simulink model "Pneumatic_act_PID"  (R2018b)
settings: Solver=ode15s  StartTime=0.0  StopTime=2  RelTol=5e-3
PreLoadFcn:
  | pneumaticInitialization
  | parametersMultibody
values from neighbouring files (symbols this model uses):
  base_breadth = 1    [parametersMultibody.m]
  base_height = 0.05    [parametersMultibody.m]
  base_length = 3.5    [parametersMultibody.m]
  box_breadth = 0.03    [parametersMultibody.m]
  box_height = 0.005    [parametersMultibody.m]
  box_height_s = 0.002    [parametersMultibody.m]
  box_length = 0.03    [parametersMultibody.m]
  box_yellow_breadth = 0.3    [parametersMultibody.m]
  box_yellow_height = 0.02    [parametersMultibody.m]
  box_yellow_length = 0.2    [parametersMultibody.m]
  frame_stand_breadth = 0.02    [parametersMultibody.m]
  frame_stand_height = 0.4280    (= 0.428)    [parametersMultibody.m]
  frame_stand_length = 0.02    [parametersMultibody.m]
undefined symbols (not defined in the file or in its folder): A_pipe, A_piston, delta_p, L_pipe, L_piston, p_init, sigbuilder_block, T_init, X, Y, Z
libraries: sm_lib x51, fl_lib x33, Contact_Forces_Lib x15, nesl_utility x7, simulink x2, Multibody_Parts_Lib x2, SimscapeFluids_lib x1, sm_backhoe_lib x1
(part 3 of 4)

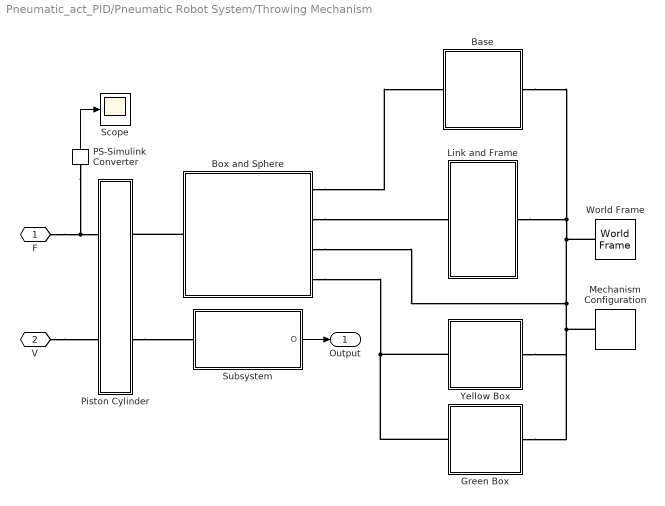
== system Pneumatic_act_PID/Pneumatic Robot System/Throwing Mechanism ==
  Base : Subsystem
      mask Display:
      | image("Base.jpg")
      | port_label('rconn', 1, 'B')
      | port_label('lconn', 1, 'W')
  Box and Sphere : Subsystem
      mask Display:
      | image('Box_ball.jpg')
      | port_label('rconn', 1, 'L')
      | port_label('lconn', 1, 'Base')
      | port_label('lconn', 2, 'Link_port')
      | port_label('lconn', 3, 'T')
      | port_label('lconn', 4, 'Ball_port')
  Green Box : Subsystem
      mask Display:
      | image("Box_green.jpg")
      | port_label('lconn', 1, 'BP')
      | port_label('rconn', 1, 'W')
  Link and Frame : Subsystem
      mask Display:
      | image('Frame_link.jpg')
      | port_label('rconn', 1, 'LP')
      | port_label('lconn', 1, 'T')
  Mechanism Configuration : sm_lib/Utilities/Mechanism Configuration  UniformGravity=Constant  GravityVector=[0 0 -9.80665]  GravityUnits=m/s^2  LinearizationDelta=0.001
  PS-Simulink Converter : nesl_utility/PS-Simulink Converter  PhysicalDomain=network_engine_domain  SubClassName=ps_output  LeftPortType=input  RightPortType=output  PseudoPeriodic=off  Frequencies=[]  Unit=1  AffineConversion=off
  Piston Cylinder : Subsystem
      mask Display: image('Piston_cyl.jpg')
  Scope : Scope
  Subsystem : Subsystem
  World Frame : sm_lib/Frames and Transforms/World Frame
  Yellow Box : Subsystem
      mask Display:
      | image("Box_yellow.jpg")
      | port_label('lconn', 1, 'BP')
      | port_label('rconn', 1, 'W')
  F : PMIOPort  Side=Left
  V : PMIOPort  Port=2  Side=Left
  Output : Outport
  wires:
  Subsystem/1(O) -> Output/1
  PS-Simulink Converter/1 -> Scope/1
  connections:
  Base/LConn1 -- World Frame/RConn1 -- Box and Sphere/LConn3 -- Mechanism Configuration/RConn1 -- Green Box/RConn1 -- Yellow Box/RConn1 -- Link and Frame/LConn1
  Box and Sphere/RConn1 -- Piston Cylinder/RConn1
  Green Box/LConn1 -- Box and Sphere/LConn4 -- Yellow Box/LConn1
  Box and Sphere/LConn2 -- Link and Frame/RConn1
  Box and Sphere/LConn1 -- Base/RConn1
  Piston Cylinder/RConn2 -- Subsystem/LConn1
  F/RConn1 -- Piston Cylinder/LConn1 -- PS-Simulink Converter/LConn1
  V/RConn1 -- Piston Cylinder/LConn2

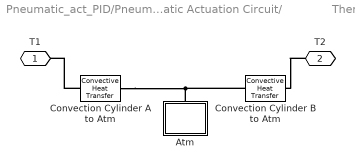
== system Pneumatic_act_PID/Pneumatic Robot System/Pneumatic Actuation Circuit/               Thermal Connection_3  ==
  Atm : Subsystem
      mask Display: disp('Atm')
  Convection Cylinder A to Atm : fl_lib/Thermal/Thermal Elements/Convective Heat Transfer  area=2*A_piston + sqrt(pi*A_piston)*L_piston m^2  heat_tr_coeff=20 W/(m^2 * K)  T_specify=off  T_priority=None  T=0 K  T_nominal_specify=off  T_nominal_unit=K  T_nominal_value=1  Q_specify=off  Q_priority=None  Q=0 W  Q_nominal_specify=off  Q_nominal_unit=W  Q_nominal_value=1
  Convection Cylinder B to Atm : fl_lib/Thermal/Thermal Elements/Convective Heat Transfer  area=2*A_piston + sqrt(pi*A_piston)*L_piston m^2  heat_tr_coeff=20 W/(m^2 * K)  T_specify=off  T_priority=None  T=0 K  T_nominal_specify=off  T_nominal_unit=K  T_nominal_value=1  Q_specify=off  Q_priority=None  Q=0 W  Q_nominal_specify=off  Q_nominal_unit=W  Q_nominal_value=1
  T1 : PMIOPort  Side=Left
  T2 : PMIOPort  Port=2  Side=Left
  connections:
  Convection Cylinder A to Atm/RConn1 -- Convection Cylinder B to Atm/RConn1 -- Atm/RConn1
  Convection Cylinder A to Atm/LConn1 -- T1/RConn1
  T2/RConn1 -- Convection Cylinder B to Atm/LConn1

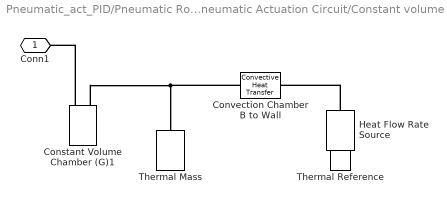
== system Pneumatic_act_PID/Pneumatic Robot System/Pneumatic Actuation Circuit/Constant volume chamber ==
  Constant Volume Chamber (G)1 : fl_lib/Gas/Elements/Constant Volume Chamber (G)  volume=volume m^3  area_A=area_A m^2  p_chamber_specify=on  p_chamber_priority=High  p_chamber=p_chamber MPa  p_chamber_nominal_specify=off  p_chamber_nominal_unit=MPa  p_chamber_nominal_value=1  T_chamber_specify=off  T_chamber_priority=High  T_chamber=293.15 K  T_chamber_nominal_specify=off  T_chamber_nominal_unit=K  T_chamber_nominal_value=1  rho_chamber_specify=off  rho_chamber_priority=None  rho_chamber=1.2 kg/m^3  rho_chamber_nominal_specify=off  rho_chamber_nominal_unit=kg/m^3  rho_chamber_nominal_value=1
      settings: SourceProductName=Simscape  SourceProductBaseCode=SS
  Convection Chamber B to Wall : fl_lib/Thermal/Thermal Elements/Convective Heat Transfer  area=area m^2  heat_tr_coeff=heat_tr_coeff W/(m^2 * K)  T_specify=off  T_priority=None  T=0 K  T_nominal_specify=off  T_nominal_unit=K  T_nominal_value=1  Q_specify=off  Q_priority=None  Q=0 W  Q_nominal_specify=off  Q_nominal_unit=W  Q_nominal_value=1
  Heat Flow Rate Source : fl_lib/Thermal/Thermal Sources/Heat Flow Rate Source  heat_flow=heat_flow W
      settings: SourceProductName=Simscape  SourceProductBaseCode=SS
  Thermal Mass : fl_lib/Thermal/Thermal Elements/Thermal Mass  mass=0.214 kg  sp_heat=840 J/kg/K  T_specify=on  T_priority=Low  T=293.15 K  T_nominal_specify=off  T_nominal_unit=K  T_nominal_value=1  Q_specify=off  Q_priority=None  Q=0 W  Q_nominal_specify=off  Q_nominal_unit=W  Q_nominal_value=1
  Thermal Reference : fl_lib/Thermal/Thermal Elements/Thermal Reference
  Conn1 : PMIOPort  Side=Left
  connections:
  Heat Flow Rate Source/LConn1 -- Convection Chamber B to Wall/LConn1
  Constant Volume Chamber (G)1/LConn2 -- Convection Chamber B to Wall/RConn1 -- Thermal Mass/LConn1
  Constant Volume Chamber (G)1/LConn1 -- Conn1/RConn1
  Thermal Reference/LConn1 -- Heat Flow Rate Source/RConn1

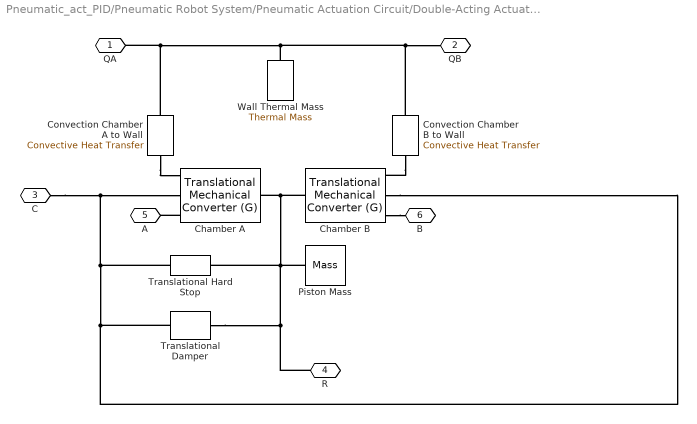
== system Pneumatic_act_PID/Pneumatic Robot System/Pneumatic Actuation Circuit/Double-Acting Actuator ==
  Chamber A : fl_lib/Gas/Elements/Translational Mechanical Converter (G)  mech_orientation=1  interface_area=A_piston m^2  length_init=x_init m  dead_volume=0.1 * A_piston * x_max m^3  area_A=A_port m^2  environment_spec=1  environment_pressure=0.101325 MPa  p_converter_specify=on  p_converter_priority=High  p_converter=p_init MPa  p_converter_nominal_specify=off  p_converter_nominal_unit=MPa  p_converter_nominal_value=1  T_converter_specify=on  T_converter_priority=High  T_converter=T_init K  T_converter_nominal_specify=off  T_converter_nominal_unit=K  T_converter_nominal_value=1  rho_converter_specify=off  rho_converter_priority=None  rho_converter=1.2 kg/m^3  rho_converter_nominal_specify=off  rho_converter_nominal_unit=kg/m^3  rho_converter_nominal_value=1
      settings: SourceProductName=Simscape  SourceProductBaseCode=SS
  Chamber B : fl_lib/Gas/Elements/Translational Mechanical Converter (G)  mech_orientation=-1  interface_area=A_piston m^2  length_init=- x_max + x_init m  dead_volume=0.1 * A_piston * x_max m^3  area_A=A_port m^2  environment_spec=1  environment_pressure=0.101325 MPa  p_converter_specify=on  p_converter_priority=High  p_converter=p_init MPa  p_converter_nominal_specify=off  p_converter_nominal_unit=MPa  p_converter_nominal_value=1  T_converter_specify=on  T_converter_priority=High  T_converter=T_init K  T_converter_nominal_specify=off  T_converter_nominal_unit=K  T_converter_nominal_value=1  rho_converter_specify=off  rho_converter_priority=None  rho_converter=1.2 kg/m^3  rho_converter_nominal_specify=off  rho_converter_nominal_unit=kg/m^3  rho_converter_nominal_value=1
      settings: SourceProductName=Simscape  SourceProductBaseCode=SS
  Convection Chamber A to Wall : fl_lib/Thermal/Thermal Elements/Convective Heat Transfer  area=2*A_piston + sqrt(pi*A_piston)*x_max m^2  heat_tr_coeff=heat_coeff W/(m^2 * K)  T_specify=off  T_priority=None  T=0 K  T_nominal_specify=off  T_nominal_unit=K  T_nominal_value=1  Q_specify=off  Q_priority=None  Q=0 W  Q_nominal_specify=off  Q_nominal_unit=W  Q_nominal_value=1
  Convection Chamber B to Wall : fl_lib/Thermal/Thermal Elements/Convective Heat Transfer  area=2*A_piston + sqrt(pi*A_piston)*x_max m^2  heat_tr_coeff=heat_coeff W/(m^2 * K)  T_specify=off  T_priority=None  T=0 K  T_nominal_specify=off  T_nominal_unit=K  T_nominal_value=1  Q_specify=off  Q_priority=None  Q=0 W  Q_nominal_specify=off  Q_nominal_unit=W  Q_nominal_value=1
  Piston Mass : fl_lib/Mechanical/Translational Elements/Mass  mass=M_piston kg  v_specify=off  v_priority=High  v=0 m/s  v_nominal_specify=off  v_nominal_unit=m/s  v_nominal_value=1  f_specify=off  f_priority=None  f=0 N  f_nominal_specify=off  f_nominal_unit=N  f_nominal_value=1
  Translational Damper : fl_lib/Mechanical/Translational Elements/Translational Damper  D=damp_mech N/(m/s)  v_specify=off  v_priority=None  v=0 m/s  v_nominal_specify=off  v_nominal_unit=m/s  v_nominal_value=1  f_specify=off  f_priority=None  f=0 N  f_nominal_specify=off  f_nominal_unit=N  f_nominal_value=1
  Translational Hard Stop : fl_lib/Mechanical/Translational Elements/Translational Hard Stop  upper_bnd=x_max m  lower_bnd=0 m  stiff_up=stiff_hard_stop N/m  stiff_low=stiff_hard_stop N/m  D_up=damp_hard_stop N/(m/s)  D_low=damp_hard_stop N/(m/s)  model=3  transition=0.1 mm  v_specify=off  v_priority=None  v=0 m/s  v_nominal_specify=off  v_nominal_unit=m/s  v_nominal_value=1  f_specify=off  f_priority=None  f=0 N  f_nominal_specify=off  f_nominal_unit=N  f_nominal_value=1  x_specify=on  x_priority=High  x=x_init m  x_nominal_specify=off  x_nominal_unit=m  x_nominal_value=1
  Wall Thermal Mass : fl_lib/Thermal/Thermal Elements/Thermal Mass  mass=M_actuator kg  sp_heat=cp J/kg/K  T_specify=on  T_priority=High  T=T_init K  T_nominal_specify=off  T_nominal_unit=K  T_nominal_value=1  Q_specify=off  Q_priority=None  Q=0 W  Q_nominal_specify=off  Q_nominal_unit=W  Q_nominal_value=1
  QA : PMIOPort  Side=Left
  QB : PMIOPort  Port=2  Side=Right
  C : PMIOPort  Port=3  Side=Left
  R : PMIOPort  Port=4  Side=Right
  A : PMIOPort  Port=5  Side=Left
  B : PMIOPort  Port=6  Side=Right
  connections:
  Chamber B/RConn1 -- R/RConn1 -- Translational Damper/LConn1 -- Piston Mass/LConn1 -- Translational Hard Stop/LConn1 -- Chamber A/RConn1
  Convection Chamber A to Wall/RConn1 -- QA/RConn1 -- Wall Thermal Mass/LConn1 -- Convection Chamber B to Wall/RConn1 -- QB/RConn1
  Translational Hard Stop/RConn1 -- Chamber B/LConn2 -- Translational Damper/RConn1 -- C/RConn1 -- Chamber A/LConn2
  Chamber A/LConn1 -- A/RConn1
  Chamber B/LConn1 -- B/RConn1
  Convection Chamber A to Wall/LConn1 -- Chamber A/LConn3
  Convection Chamber B to Wall/LConn1 -- Chamber B/LConn3

== system Pneumatic_act_PID/Pneumatic Robot System/Pneumatic Actuation Circuit/Pipe A ==
  Pipe (G) : fl_lib/Gas/Elements/Pipe (G)  length=L_pipe m  area=A_pipe m^2  Dh=2*sqrt(A_pipe/pi) m  length_add=0.1 * L_pipe m  roughness=15e-6 m  Re_lam=2000  Re_tur=4000  shape_factor=64  Nu_lam=3.66  p_pipe_specify=on  p_pipe_priority=Low  p_pipe=0.101325 MPa  p_pipe_nominal_specify=off  p_pipe_nominal_unit=MPa  p_pipe_nominal_value=1  T_pipe_specify=on  T_pipe_priority=Low  T_pipe=293.15 K  T_pipe_nominal_specify=off  T_pipe_nominal_unit=K  T_pipe_nominal_value=1  rho_pipe_specify=on  rho_pipe_priority=Low  rho_pipe=1.2 kg/m^3  rho_pipe_nominal_specify=off  rho_pipe_nominal_unit=kg/m^3  rho_pipe_nominal_value=1
      settings: SourceProductName=Simscape  SourceProductBaseCode=SS
  Wall Thermal Mass : fl_lib/Thermal/Thermal Elements/Thermal Mass  mass=rho_wall * A_pipe * L_pipe kg  sp_heat=cp_wall J/kg/K  T_specify=off  T_priority=High  T=T_init K  T_nominal_specify=off  T_nominal_unit=K  T_nominal_value=1  Q_specify=off  Q_priority=None  Q=0 W  Q_nominal_specify=off  Q_nominal_unit=W  Q_nominal_value=1
  B : PMIOPort  Side=Right
  A : PMIOPort  Port=2  Side=Left
  T : PMIOPort  Port=3  Side=Left
  connections:
  Pipe (G)/RConn1 -- B/RConn1
  A/RConn1 -- Pipe (G)/LConn1
  Pipe (G)/LConn2 -- Wall Thermal Mass/LConn1 -- T/RConn1

== system Pneumatic_act_PID/Pneumatic Robot System/Pneumatic Actuation Circuit/Pipe B ==
  Pipe (G) : fl_lib/Gas/Elements/Pipe (G)  length=L_pipe m  area=A_pipe m^2  Dh=2*sqrt(A_pipe/pi) m  length_add=0.1 * L_pipe m  roughness=15e-6 m  Re_lam=2000  Re_tur=4000  shape_factor=64  Nu_lam=3.66  p_pipe_specify=on  p_pipe_priority=Low  p_pipe=0.101325 MPa  p_pipe_nominal_specify=off  p_pipe_nominal_unit=MPa  p_pipe_nominal_value=1  T_pipe_specify=on  T_pipe_priority=Low  T_pipe=293.15 K  T_pipe_nominal_specify=off  T_pipe_nominal_unit=K  T_pipe_nominal_value=1  rho_pipe_specify=on  rho_pipe_priority=Low  rho_pipe=1.2 kg/m^3  rho_pipe_nominal_specify=off  rho_pipe_nominal_unit=kg/m^3  rho_pipe_nominal_value=1
      settings: SourceProductName=Simscape  SourceProductBaseCode=SS
  Wall Thermal Mass : fl_lib/Thermal/Thermal Elements/Thermal Mass  mass=rho_wall * A_pipe * L_pipe kg  sp_heat=cp_wall J/kg/K  T_specify=off  T_priority=High  T=T_init K  T_nominal_specify=off  T_nominal_unit=K  T_nominal_value=1  Q_specify=off  Q_priority=None  Q=0 W  Q_nominal_specify=off  Q_nominal_unit=W  Q_nominal_value=1
  B : PMIOPort  Side=Right
  T : PMIOPort  Port=2  Side=Left
  A : PMIOPort  Port=3  Side=Left
  connections:
  T/RConn1 -- Wall Thermal Mass/LConn1 -- Pipe (G)/LConn2
  A/RConn1 -- Pipe (G)/LConn1
  Pipe (G)/RConn1 -- B/RConn1

== system Pneumatic_act_PID/Pneumatic Robot System/Pneumatic Actuation Circuit/Return Pipe ==
  Pipe (G) : fl_lib/Gas/Elements/Pipe (G)  length=L_pipe m  area=A_pipe m^2  Dh=2*sqrt(A_pipe/pi) m  length_add=0.1 * L_pipe m  roughness=15e-6 m  Re_lam=2000  Re_tur=4000  shape_factor=64  Nu_lam=3.66  p_pipe_specify=off  p_pipe_priority=Low  p_pipe=0.101325 MPa  p_pipe_nominal_specify=off  p_pipe_nominal_unit=MPa  p_pipe_nominal_value=1  T_pipe_specify=off  T_pipe_priority=Low  T_pipe=293.15 K  T_pipe_nominal_specify=off  T_pipe_nominal_unit=K  T_pipe_nominal_value=1  rho_pipe_specify=off  rho_pipe_priority=Low  rho_pipe=1.2 kg/m^3  rho_pipe_nominal_specify=off  rho_pipe_nominal_unit=kg/m^3  rho_pipe_nominal_value=1
      settings: SourceProductName=Simscape  SourceProductBaseCode=SS
  Wall Thermal Mass : fl_lib/Thermal/Thermal Elements/Thermal Mass  mass=rho_wall * A_pipe * L_pipe kg  sp_heat=cp_wall J/kg/K  T_specify=off  T_priority=None  T=300 K  T_nominal_specify=off  T_nominal_unit=K  T_nominal_value=1  Q_specify=off  Q_priority=None  Q=0 W  Q_nominal_specify=off  Q_nominal_unit=W  Q_nominal_value=1
  B : PMIOPort  Side=Right
  T : PMIOPort  Port=2  Side=Left
  A : PMIOPort  Port=3  Side=Left
  connections:
  Pipe (G)/RConn1 -- B/RConn1
  A/RConn1 -- Pipe (G)/LConn1
  Pipe (G)/LConn2 -- Wall Thermal Mass/LConn1 -- T/RConn1

== system Pneumatic_act_PID/Pneumatic Robot System/Pneumatic Actuation Circuit/Supply Pipe ==
  Pipe (G) : fl_lib/Gas/Elements/Pipe (G)  length=L_pipe m  area=A_pipe m^2  Dh=2*sqrt(A_pipe/pi) m  length_add=0.1 * L_pipe m  roughness=15e-6 m  Re_lam=2000  Re_tur=4000  shape_factor=64  Nu_lam=3.66  p_pipe_specify=on  p_pipe_priority=Low  p_pipe=0.101325 MPa  p_pipe_nominal_specify=off  p_pipe_nominal_unit=MPa  p_pipe_nominal_value=1  T_pipe_specify=on  T_pipe_priority=Low  T_pipe=293.15 K  T_pipe_nominal_specify=off  T_pipe_nominal_unit=K  T_pipe_nominal_value=1  rho_pipe_specify=on  rho_pipe_priority=Low  rho_pipe=1.2 kg/m^3  rho_pipe_nominal_specify=off  rho_pipe_nominal_unit=kg/m^3  rho_pipe_nominal_value=1
      settings: SourceProductName=Simscape  SourceProductBaseCode=SS
  Wall Thermal Mass : fl_lib/Thermal/Thermal Elements/Thermal Mass  mass=rho_wall * A_pipe * L_pipe kg  sp_heat=cp_wall J/kg/K  T_specify=off  T_priority=Low  T=T_init K  T_nominal_specify=off  T_nominal_unit=K  T_nominal_value=1  Q_specify=off  Q_priority=None  Q=0 W  Q_nominal_specify=off  Q_nominal_unit=W  Q_nominal_value=1
  B : PMIOPort  Side=Right
  A : PMIOPort  Port=2  Side=Left
  T : PMIOPort  Port=3  Side=Left
  connections:
  T/RConn1 -- Wall Thermal Mass/LConn1 -- Pipe (G)/LConn2
  A/RConn1 -- Pipe (G)/LConn1
  Pipe (G)/RConn1 -- B/RConn1

== system Pneumatic_act_PID/Pneumatic Robot System/Pneumatic Actuation Circuit/Thermal Connection_1 ==
  Atm2 : Subsystem
      mask Display: disp('Atm')
  Convection Return to Atm : fl_lib/Thermal/Thermal Elements/Convective Heat Transfer  area=2*sqrt(pi*A_pipe) * L_pipe m^2  heat_tr_coeff=20 W/(m^2 * K)  T_specify=off  T_priority=None  T=0 K  T_nominal_specify=off  T_nominal_unit=K  T_nominal_value=1  Q_specify=off  Q_priority=None  Q=0 W  Q_nominal_specify=off  Q_nominal_unit=W  Q_nominal_value=1
  Convection Supply to Atm : fl_lib/Thermal/Thermal Elements/Convective Heat Transfer  area=2*sqrt(pi*A_pipe) * L_pipe m^2  heat_tr_coeff=20 W/(m^2 * K)  T_specify=off  T_priority=None  T=0 K  T_nominal_specify=off  T_nominal_unit=K  T_nominal_value=1  Q_specify=off  Q_priority=None  Q=0 W  Q_nominal_specify=off  Q_nominal_unit=W  Q_nominal_value=1
  T1 : PMIOPort  Side=Left
  T2 : PMIOPort  Port=2  Side=Left
  connections:
  Convection Supply to Atm/LConn1 -- T1/RConn1
  Convection Return to Atm/RConn1 -- Convection Supply to Atm/RConn1 -- Atm2/RConn1
  Convection Return to Atm/LConn1 -- T2/RConn1

== system Pneumatic_act_PID/Pneumatic Robot System/Pneumatic Actuation Circuit/Thermal Connection_2 ==
  Atm1 : Subsystem
      mask Display: disp('Atm')
  Convection Pipe A to Atm : fl_lib/Thermal/Thermal Elements/Convective Heat Transfer  area=2*sqrt(pi*A_pipe) * L_pipe m^2  heat_tr_coeff=20 W/(m^2 * K)  T_specify=off  T_priority=None  T=0 K  T_nominal_specify=off  T_nominal_unit=K  T_nominal_value=1  Q_specify=off  Q_priority=None  Q=0 W  Q_nominal_specify=off  Q_nominal_unit=W  Q_nominal_value=1
  Convection Pipe B to Atm : fl_lib/Thermal/Thermal Elements/Convective Heat Transfer  area=2*sqrt(pi*A_pipe) * L_pipe m^2  heat_tr_coeff=20 W/(m^2 * K)  T_specify=off  T_priority=None  T=0 K  T_nominal_specify=off  T_nominal_unit=K  T_nominal_value=1  Q_specify=off  Q_priority=None  Q=0 W  Q_nominal_specify=off  Q_nominal_unit=W  Q_nominal_value=1
  T1 : PMIOPort  Side=Left
  T2 : PMIOPort  Port=2  Side=Left
  connections:
  Convection Pipe B to Atm/RConn1 -- Convection Pipe A to Atm/RConn1 -- Atm1/RConn1
  Convection Pipe A to Atm/LConn1 -- T1/RConn1
  Convection Pipe B to Atm/LConn1 -- T2/RConn1

== system Pneumatic_act_PID/Pneumatic Robot System/Throwing Mechanism/Base ==
  " Base" : sm_lib/Body Elements/Solid  InertiaType=CalculateFromGeometry  Mass=1  MassUnits=kg  CenterOfMass=[0 0 0]  CenterOfMassUnits=m  MomentsOfInertia=[1 1 1]  MomentsOfInertiaUnits=kg*m^2  ProductsOfInertia=[0 0 0]  ProductsOfInertiaUnits=kg*m^2  BasedOnType=Density  Density=1000  DensityUnits=kg/m^3  DoExposeReferenceFrame=on  SerializedFrames=<Frames/>  GraphicType=FromGeometry  MarkerShape=Sphere  MarkerSize=10  GraphicVisPropType=SimpleVisualProperties  GraphicDiffuseColor=[0.8 1 0.8]  GraphicSpecularColor=[0.5 0.5 0.5 1.0]  GraphicAmbientColor=[0.15 0.15 0.15 1.0]  GraphicEmissiveColor=[0.0 0.0 0.0 1.0]  GraphicShininess=75  GraphicOpacity=1.0  GeometryShape=Brick  RectangleSize=[1 1]  RectangleSizeUnits=m  BrickDimensions=[base_length base_breadth base_height]  BrickDimensionUnits=m  CylinderRadius=0.008  CylinderRadiusUnits=m  CylinderLength=0.1  CylinderLengthUnits=m  SphereRadius=1  SphereRadiusUnits=m  EllipsoidRadii=[1 1 1]  EllipsoidRadiiUnits=m  ExtrusionCrossSection=[1 1; -1 1; -1 -1; 1 -1]  ExtrusionCrossSectionUnits=m  ExtrusionLength=1  ExtrusionLengthUnits=m  PolygonNumSides=3  PolygonOuterRadius=1  PolygonOuterRadiusUnits=m  ExtGeomFileType=STEP  ExtGeomFileUnits=m  RevolutionCrossSection=[1 1; 1 -1; 2 -1; 2 1]  RevolutionCrossSectionUnits=m  RevolutionExtent=Full  RevolutionAngle=180  RevolutionAngleUnits=deg
  Rigid Transform3 : sm_lib/Frames and Transforms/Rigid Transform  TranslationMethod=Cartesian  TranslationStandardOffset=0.25  TranslationLengthUnit=m  TranslationStandardAxis=-Z  TranslationCartesianOffset=[1.2 0 -0.25]  TranslationROffset=0  TranslationROffsetUnits=m  TranslationZOffset=0  TranslationZOffsetUnits=m  TranslationThetaOffset=0  TranslationThetaOffsetUnits=deg  RotationMethod=None  RotationAngleUnits=deg  RotationStandardAxis=+X  RotationAngle=90  RotationArbitraryAxis=[0 0 1]  FollAlignAxisA=+X  BaseAlignAxisA=+Y  FollAlignAxisB=+Y  BaseAlignAxisB=+Z  RotationSequenceAxes=FollowerAxes  RotationSequence=XYX  RotationSequenceAngles=[0 0 0]  RotationSequenceAnglesUnits=deg  RotationMatrix=[1 0 0; 0 1 0; 0 0 1]
  B : PMIOPort  Side=Left
  Base : PMIOPort  Port=2  Side=Right
  connections:
  Rigid Transform3/RConn1 -- Base/RConn1 -- " Base"/RConn1
  Rigid Transform3/LConn1 -- B/RConn1

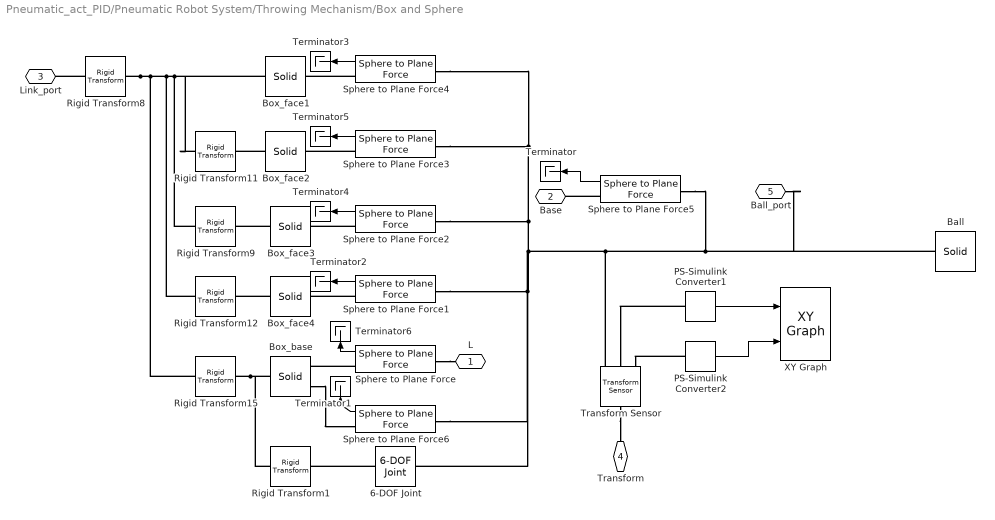
== system Pneumatic_act_PID/Pneumatic Robot System/Throwing Mechanism/Box and Sphere ==
  6-DOF Joint : sm_lib/Joints/6-DOF Joint  SenseConstraintForce=off  SenseConstraintForceX=off  SenseConstraintForceY=off  SenseConstraintForceZ=off  SenseConstraintTorque=off  SenseConstraintTorqueX=off  SenseConstraintTorqueY=off  SenseConstraintTorqueZ=off  SenseTotalForce=off  SenseTotalForceX=off  SenseTotalForceY=off  SenseTotalForceZ=off  SenseTotalTorque=off  SenseTotalTorqueX=off  SenseTotalTorqueY=off  SenseTotalTorqueZ=off  CompositeWrenchDir=FollowerOnBase  CompositeWrenchFrame=BaseFrame  PxEquilibriumPosition=0  PxEquilibriumPositionUnits=m  PxSpringStiffness=0  PxSpringStiffnessUnits=N/m  PxDampingCoefficient=0  PxDampingCoefficientUnits=N/(m/s)  PxTorqueActuationMode=NoTorque  PxMotionActuationMode=ComputedMotion  PxSensePosition=off  PxSenseVelocity=off  PxSenseAcceleration=off  PxSenseTorqueForce=off  PxPositionTargetSpecify=off  PxPositionTargetPriority=High  PxPositionTargetValue=0  PxPositionTargetValueUnits=m  PxVelocityTargetSpecify=off  PxVelocityTargetPriority=High  PxVelocityTargetValue=0  PxVelocityTargetValueUnits=m/s  PyEquilibriumPosition=0  PyEquilibriumPositionUnits=m  PySpringStiffness=0  PySpringStiffnessUnits=N/m  PyDampingCoefficient=0  PyDampingCoefficientUnits=N/(m/s)  PyTorqueActuationMode=NoTorque  PyMotionActuationMode=ComputedMotion  PySensePosition=off  PySenseVelocity=off  PySenseAcceleration=off  PySenseTorqueForce=off  PyPositionTargetSpecify=off  PyPositionTargetPriority=High  PyPositionTargetValue=0  PyPositionTargetValueUnits=m  PyVelocityTargetSpecify=off  PyVelocityTargetPriority=High  PyVelocityTargetValue=0  PyVelocityTargetValueUnits=m/s  PzEquilibriumPosition=0  PzEquilibriumPositionUnits=m  PzSpringStiffness=0  PzSpringStiffnessUnits=N/m  PzDampingCoefficient=0  PzDampingCoefficientUnits=N/(m/s)  PzTorqueActuationMode=NoTorque  PzMotionActuationMode=ComputedMotion  PzSensePosition=off  PzSenseVelocity=off  PzSenseAcceleration=off  PzSenseTorqueForce=off  PzPositionTargetSpecify=off  PzPositionTargetPriority=High  PzPositionTargetValue=0  PzPositionTargetValueUnits=m  PzVelocityTargetSpecify=off  PzVelocityTargetPriority=High  PzVelocityTargetValue=0  PzVelocityTargetValueUnits=m/s  SphDefPosRotationMethod=None  SphDefPosRotationAngleUnits=deg  SphDefPosRotationStandardAxis=+Z  SphDefPosRotationAngle=0.0  SphDefPosRotationArbitraryAxis=[0 0 1]  SphDefPosFollAlignAxisA=+X  SphDefPosBaseAlignAxisA=+Y  SphDefPosFollAlignAxisB=+Y  SphDefPosBaseAlignAxisB=+Z  SphDefPosRotationSequenceAxes=FollowerAxes  SphDefPosRotationSequence=XYX  SphDefPosRotationSequenceAngles=[0 0 0]  SphDefPosRotationSequenceAnglesUnits=deg  SphDefPosRotationMatrix=[1 0 0; 0 1 0; 0 0 1]  SphEqPosRotationMethod=None  SphEqPosRotationAngleUnits=deg  SphEqPosRotationStandardAxis=+Z  SphEqPosRotationAngle=0.0  SphEqPosRotationArbitraryAxis=[0 0 1]  SphEqPosFollAlignAxisA=+X  SphEqPosBaseAlignAxisA=+Y  SphEqPosFollAlignAxisB=+Y  SphEqPosBaseAlignAxisB=+Z  SphEqPosRotationSequenceAxes=FollowerAxes  SphEqPosRotationSequence=XYX  SphEqPosRotationSequenceAngles=[0 0 0]  SphEqPosRotationSequenceAnglesUnits=deg  SphEqPosRotationMatrix=[1 0 0; 0 1 0; 0 0 1]  SphSpringStiffness=0  SphSpringStiffnessUnits=N*m/deg  SphDampingCoefficient=1e-3  SphDampingCoefficientUnits=N*m/(rad/s)  SphActuateTorqueX=off  SphActuateTorqueY=off  SphActuateTorqueZ=off  SphActuateTorque=off  SphTorqueActuationMode=NoTorque  SphMotionActuationMode=ComputedMotion  SphActuationFrame=BaseFrame  SphSensePosition=off  SphSenseVelocityX=off  SphSenseVelocityY=off  SphSenseVelocityZ=off  SphSenseVelocity=off  SphSenseAccelerationX=off  SphSenseAccelerationY=off  SphSenseAccelerationZ=off  SphSenseAcceleration=off  SphSenseTorqueX=off  SphSenseTorqueY=off  SphSenseTorqueZ=off  SphSenseTorqueForce=off  SphSensingFrame=BaseFrame  SphPositionTargetRotationMethod=None  SphPositionTargetRotationAngleUnits=deg  SphPositionTargetRotationStandardAxis=+Z  SphPositionTargetRotationAngle=0.0  SphPositionTargetRotationArbitraryAxis=[0 0 1]  SphPositionTargetFollAlignAxisA=+X  SphPositionTargetBaseAlignAxisA=+Y  SphPositionTargetFollAlignAxisB=+Y  SphPositionTargetBaseAlignAxisB=+Z  SphPositionTargetRotationSequenceAxes=FollowerAxes  SphPositionTargetRotationSequence=XYX  SphPositionTargetRotationSequenceAngles=[0 0 0]  SphPositionTargetRotationSequenceAnglesUnits=deg  SphPositionTargetRotationMatrix=[1 0 0; 0 1 0; 0 0 1]  SphPositionTargetSpecify=off  SphPositionTargetPriority=High  SphVelocityTargetValue=[0 0 0]  SphVelocityTargetValueUnits=deg/s  SphVelocityTargetSpecify=off  SphVelocityTargetPriority=High  SphVelocityTargetInFollowerFrame=on
  Ball : sm_lib/Body Elements/Solid  InertiaType=CalculateFromGeometry  Mass=15  MassUnits=g  CenterOfMass=[0 0 0]  CenterOfMassUnits=m  MomentsOfInertia=[1 1 1]  MomentsOfInertiaUnits=kg*m^2  ProductsOfInertia=[0 0 0]  ProductsOfInertiaUnits=kg*m^2  BasedOnType=Density  Density=1000  DensityUnits=kg/m^3  DoExposeReferenceFrame=on  SerializedFrames=<Frames/>  GraphicType=FromGeometry  MarkerShape=Sphere  MarkerSize=10  GraphicVisPropType=SimpleVisualProperties  GraphicDiffuseColor=[1 1 0.4]  GraphicSpecularColor=[0.5 0.5 0.5 1.0]  GraphicAmbientColor=[0.15 0.15 0.15 1.0]  GraphicEmissiveColor=[0.0 0.0 0.0 1.0]  GraphicShininess=75  GraphicOpacity=1.0  GeometryShape=Sphere  RectangleSize=[1 1]  RectangleSizeUnits=m  BrickDimensions=[1 1 1]  BrickDimensionUnits=m  CylinderRadius=1  CylinderRadiusUnits=m  CylinderLength=1  CylinderLengthUnits=m  SphereRadius=radius_ball  SphereRadiusUnits=m  EllipsoidRadii=[1 1 1]  EllipsoidRadiiUnits=m  ExtrusionCrossSection=[1 1; -1 1; -1 -1; 1 -1]  ExtrusionCrossSectionUnits=m  ExtrusionLength=1  ExtrusionLengthUnits=m  PolygonNumSides=3  PolygonOuterRadius=1  PolygonOuterRadiusUnits=m  ExtGeomFileType=STEP  ExtGeomFileUnits=m  RevolutionCrossSection=[1 1; 1 -1; 2 -1; 2 1]  RevolutionCrossSectionUnits=m  RevolutionExtent=Full  RevolutionAngle=180  RevolutionAngleUnits=deg
  Box_base : sm_lib/Body Elements/Solid  InertiaType=CalculateFromGeometry  Mass=1  MassUnits=kg  CenterOfMass=[0 0 0]  CenterOfMassUnits=m  MomentsOfInertia=[1 1 1]  MomentsOfInertiaUnits=kg*m^2  ProductsOfInertia=[0 0 0]  ProductsOfInertiaUnits=kg*m^2  BasedOnType=Density  Density=1000  DensityUnits=kg/m^3  DoExposeReferenceFrame=on  SerializedFrames=<Frames><Frame><Id>Frame1</Id><Value><Name>F1</Name><Origin><Source>ReferenceFrame</Source><FeatureName></FeatureName></Origin><PrimaryAxis><DefinedDirection>+Z</DefinedDirection><Source>ReferenceFrame</Source><SourceDirection>+Z</SourceDirection><FeatureName></FeatureName></PrimaryAxis><SecondaryAxis><DefinedDirection>+Y</DefinedDirection><Source>ReferenceFrame</Source><SourceDirection>-X</SourceDirection><FeatureName></FeatureName></SecondaryAxis></Value></Frame><Frame><Id>Frame2</Id><Value><Name>F2</Name><Origin><Source>ReferenceFrame</Source><FeatureName></FeatureName></Origin><PrimaryAxis><DefinedDirection>+Z</DefinedDirection><Source>ReferenceFrame</Source><SourceDirection>+Z</SourceDirection><FeatureName></FeatureName></PrimaryAxis><SecondaryAxis><DefinedDirection>+X</DefinedDirection><Source>ReferenceFrame</Source><SourceDirection>+X</SourceDirection><FeatureName></FeatureName></SecondaryAxis></Value></Frame></Frames>  GraphicType=FromGeometry  MarkerShape=Sphere  MarkerSize=10  GraphicVisPropType=SimpleVisualProperties  GraphicDiffuseColor=[1.0 0.2 0.0]  GraphicSpecularColor=[0.5 0.5 0.5 1.0]  GraphicAmbientColor=[0.15 0.15 0.15 1.0]  GraphicEmissiveColor=[0.0 0.0 0.0 1.0]  GraphicShininess=75  GraphicOpacity=1  GeometryShape=Brick  RectangleSize=[1 1]  RectangleSizeUnits=m  BrickDimensions=[box_length box_breadth box_height]  BrickDimensionUnits=m  CylinderRadius=1  CylinderRadiusUnits=m  CylinderLength=1  CylinderLengthUnits=m  SphereRadius=1  SphereRadiusUnits=m  EllipsoidRadii=[1 1 1]  EllipsoidRadiiUnits=m  ExtrusionCrossSection=[1 1; -1 1; -1 -1; 1 -1]  ExtrusionCrossSectionUnits=m  ExtrusionLength=1  ExtrusionLengthUnits=m  PolygonNumSides=3  PolygonOuterRadius=1  PolygonOuterRadiusUnits=m  ExtGeomFileType=STEP  ExtGeomFileUnits=m  RevolutionCrossSection=[1 1; 1 -1; 2 -1; 2 1]  RevolutionCrossSectionUnits=m  RevolutionExtent=Full  RevolutionAngle=180  RevolutionAngleUnits=deg
  Box_face{1..4} (4 alike) : sm_lib/Body Elements/Solid  InertiaType=CalculateFromGeometry  Mass=1  MassUnits=kg  CenterOfMass=[0 0 0]  CenterOfMassUnits=m  MomentsOfInertia=[1 1 1]  MomentsOfInertiaUnits=kg*m^2  ProductsOfInertia=[0 0 0]  ProductsOfInertiaUnits=kg*m^2  BasedOnType=Density  Density=1000  DensityUnits=kg/m^3  DoExposeReferenceFrame=on  SerializedFrames=<Frames><Frame><Id>Frame1</Id><Value><Name>F1</Name><Origin><Source>ReferenceFrame</Source><FeatureName></FeatureName></Origin><PrimaryAxis><DefinedDirection>+Z</DefinedDirection><Source>ReferenceFrame</Source><SourceDirection>+Z</SourceDirection><FeatureName></FeatureName></PrimaryAxis><SecondaryAxis><DefinedDirection>+X</DefinedDirection><Source>ReferenceFrame</Source><SourceDirection>+X</SourceDirection><FeatureName></FeatureName></SecondaryAxis></Value></Frame></Frames>  GraphicType=FromGeometry  MarkerShape=Sphere  MarkerSize=10  GraphicVisPropType=SimpleVisualProperties  GraphicDiffuseColor=[1.0 0.2 0.0]  GraphicSpecularColor=[0.5 0.5 0.5 1.0]  GraphicAmbientColor=[0.15 0.15 0.15 1.0]  GraphicEmissiveColor=[0.0 0.0 0.0 1.0]  GraphicShininess=75  GraphicOpacity=0.3  GeometryShape=Brick  RectangleSize=[1 1]  RectangleSizeUnits=m  BrickDimensions=[box_length box_breadth box_height_s]  BrickDimensionUnits=m  CylinderRadius=1  CylinderRadiusUnits=m  CylinderLength=1  CylinderLengthUnits=m  SphereRadius=1  SphereRadiusUnits=m  EllipsoidRadii=[1 1 1]  EllipsoidRadiiUnits=m  ExtrusionCrossSection=[1 1; -1 1; -1 -1; 1 -1]  ExtrusionCrossSectionUnits=m  ExtrusionLength=1  ExtrusionLengthUnits=m  PolygonNumSides=3  PolygonOuterRadius=1  PolygonOuterRadiusUnits=m  ExtGeomFileType=STEP  ExtGeomFileUnits=m  RevolutionCrossSection=[1 1; 1 -1; 2 -1; 2 1]  RevolutionCrossSectionUnits=m  RevolutionExtent=Full  RevolutionAngle=180  RevolutionAngleUnits=deg
  PS-Simulink Converter1 : nesl_utility/PS-Simulink Converter  PhysicalDomain=network_engine_domain  SubClassName=ps_output  LeftPortType=input  RightPortType=output  PseudoPeriodic=off  Frequencies=[]  Unit=1  AffineConversion=off
  PS-Simulink Converter2 : nesl_utility/PS-Simulink Converter  PhysicalDomain=network_engine_domain  SubClassName=ps_output  LeftPortType=input  RightPortType=output  PseudoPeriodic=off  Frequencies=[]  Unit=1  AffineConversion=off
  Rigid Transform1 : sm_lib/Frames and Transforms/Rigid Transform  TranslationMethod=StandardAxis  TranslationStandardOffset=.027/2-0.002  TranslationLengthUnit=m  TranslationStandardAxis=+Z  TranslationCartesianOffset=[0 -0.03/2 -0.03/2]  TranslationROffset=0  TranslationROffsetUnits=m  TranslationZOffset=0  TranslationZOffsetUnits=m  TranslationThetaOffset=0  TranslationThetaOffsetUnits=deg  RotationMethod=None  RotationAngleUnits=deg  RotationStandardAxis=-X  RotationAngle=90  RotationArbitraryAxis=[0 0 1]  FollAlignAxisA=+X  BaseAlignAxisA=+Y  FollAlignAxisB=+Y  BaseAlignAxisB=+Z  RotationSequenceAxes=FollowerAxes  RotationSequence=XYX  RotationSequenceAngles=[0 0 0]  RotationSequenceAnglesUnits=deg  RotationMatrix=[1 0 0; 0 1 0; 0 0 1]
  Rigid Transform11 : sm_lib/Frames and Transforms/Rigid Transform  TranslationMethod=Cartesian  TranslationStandardOffset=0  TranslationLengthUnit=m  TranslationStandardAxis=+Z  TranslationCartesianOffset=[-0.03/2 0 -0.03/2]  TranslationROffset=0  TranslationROffsetUnits=m  TranslationZOffset=0  TranslationZOffsetUnits=m  TranslationThetaOffset=0  TranslationThetaOffsetUnits=deg  RotationMethod=StandardAxis  RotationAngleUnits=deg  RotationStandardAxis=+Y  RotationAngle=90  RotationArbitraryAxis=[0 0 1]  FollAlignAxisA=+X  BaseAlignAxisA=+Y  FollAlignAxisB=+Y  BaseAlignAxisB=+Z  RotationSequenceAxes=FollowerAxes  RotationSequence=XYX  RotationSequenceAngles=[0 0 0]  RotationSequenceAnglesUnits=deg  RotationMatrix=[1 0 0; 0 1 0; 0 0 1]
  Rigid Transform12 : sm_lib/Frames and Transforms/Rigid Transform  TranslationMethod=Cartesian  TranslationStandardOffset=0  TranslationLengthUnit=m  TranslationStandardAxis=+Z  TranslationCartesianOffset=[0 0 -0.03]  TranslationROffset=0  TranslationROffsetUnits=m  TranslationZOffset=0  TranslationZOffsetUnits=m  TranslationThetaOffset=0  TranslationThetaOffsetUnits=deg  RotationMethod=None  RotationAngleUnits=deg  RotationStandardAxis=+Y  RotationAngle=90  RotationArbitraryAxis=[0 0 1]  FollAlignAxisA=+X  BaseAlignAxisA=+Y  FollAlignAxisB=+Y  BaseAlignAxisB=+Z  RotationSequenceAxes=FollowerAxes  RotationSequence=XYX  RotationSequenceAngles=[0 0 0]  RotationSequenceAnglesUnits=deg  RotationMatrix=[1 0 0; 0 1 0; 0 0 1]
  Rigid Transform15 : sm_lib/Frames and Transforms/Rigid Transform  TranslationMethod=Cartesian  TranslationStandardOffset=0  TranslationLengthUnit=m  TranslationStandardAxis=+Z  TranslationCartesianOffset=[0 -0.03/2 -0.03/2]  TranslationROffset=0  TranslationROffsetUnits=m  TranslationZOffset=0  TranslationZOffsetUnits=m  TranslationThetaOffset=0  TranslationThetaOffsetUnits=deg  RotationMethod=StandardAxis  RotationAngleUnits=deg  RotationStandardAxis=-X  RotationAngle=90  RotationArbitraryAxis=[0 0 1]  FollAlignAxisA=+X  BaseAlignAxisA=+Y  FollAlignAxisB=+Y  BaseAlignAxisB=+Z  RotationSequenceAxes=FollowerAxes  RotationSequence=XYX  RotationSequenceAngles=[0 0 0]  RotationSequenceAnglesUnits=deg  RotationMatrix=[1 0 0; 0 1 0; 0 0 1]
  Rigid Transform8 : sm_lib/Frames and Transforms/Rigid Transform  TranslationMethod=None  TranslationStandardOffset=0  TranslationLengthUnit=m  TranslationStandardAxis=+Z  TranslationCartesianOffset=[0 0 0]  TranslationROffset=0  TranslationROffsetUnits=m  TranslationZOffset=0  TranslationZOffsetUnits=m  TranslationThetaOffset=0  TranslationThetaOffsetUnits=deg  RotationMethod=StandardAxis  RotationAngleUnits=deg  RotationStandardAxis=+Y  RotationAngle=90  RotationArbitraryAxis=[0 0 1]  FollAlignAxisA=+X  BaseAlignAxisA=+Y  FollAlignAxisB=+Y  BaseAlignAxisB=+Z  RotationSequenceAxes=FollowerAxes  RotationSequence=XYX  RotationSequenceAngles=[0 0 0]  RotationSequenceAnglesUnits=deg  RotationMatrix=[1 0 0; 0 1 0; 0 0 1]
  Rigid Transform9 : sm_lib/Frames and Transforms/Rigid Transform  TranslationMethod=Cartesian  TranslationStandardOffset=0  TranslationLengthUnit=m  TranslationStandardAxis=+Z  TranslationCartesianOffset=[0.03/2 0 -0.03/2]  TranslationROffset=0  TranslationROffsetUnits=m  TranslationZOffset=0  TranslationZOffsetUnits=m  TranslationThetaOffset=0  TranslationThetaOffsetUnits=deg  RotationMethod=StandardAxis  RotationAngleUnits=deg  RotationStandardAxis=+Y  RotationAngle=90  RotationArbitraryAxis=[0 0 1]  FollAlignAxisA=+X  BaseAlignAxisA=+Y  FollAlignAxisB=+Y  BaseAlignAxisB=+Z  RotationSequenceAxes=FollowerAxes  RotationSequence=XYX  RotationSequenceAngles=[0 0 0]  RotationSequenceAnglesUnits=deg  RotationMatrix=[1 0 0; 0 1 0; 0 0 1]
  Sphere to Plane Force : Contact_Forces_Lib/3D/Sphere to Plane Force  sphere_rad=radius_sphere  plane_lenx=box_length  plane_leny=box_breadth  plane_depth=box_height/2  force_law=Linear  k_contact=1e3  b_contact=100  pen_full_damp_F=1e-4  pen_exponent=1  custom_param_1=1  custom_param_2=1  friction_law=None  mu_kinetic=0.5  mu_static=0.7  v_thr=0.01  vis_on=off  vis_opc_en=0  vis_len_plaBz=0.005  vis_clr=[0.9 0.2 0.2]  vis_opc=0.7
  Sphere to Plane Force{1..4} (4 alike) : Contact_Forces_Lib/3D/Sphere to Plane Force  sphere_rad=radius_ball  plane_lenx=box_length  plane_leny=box_breadth  plane_depth=box_height_s/2  force_law=Linear  k_contact=500  b_contact=100  pen_full_damp_F=1e-4  pen_exponent=1  custom_param_1=1  custom_param_2=1  friction_law=None  mu_kinetic=0.5  mu_static=0.7  v_thr=0.0001  vis_on=off  vis_opc_en=0  vis_len_plaBz=0.005  vis_clr=[0.9 0.2 0.2]  vis_opc=0.7
  Sphere to Plane Force5 : Contact_Forces_Lib/3D/Sphere to Plane Force  sphere_rad=0.027/3  plane_lenx=base_length  plane_leny=base_breadth  plane_depth=base_height/2  force_law=Linear  k_contact=1e3  b_contact=100  pen_full_damp_F=1e-4  pen_exponent=1  custom_param_1=1  custom_param_2=1  friction_law=None  mu_kinetic=0.5  mu_static=0.7  v_thr=0.001  vis_on=off  vis_opc_en=0  vis_len_plaBz=0.005  vis_clr=[0.9 0.2 0.2]  vis_opc=0.7
  Sphere to Plane Force6 : Contact_Forces_Lib/3D/Sphere to Plane Force  sphere_rad=radius_ball  plane_lenx=box_length  plane_leny=box_breadth  plane_depth=box_height/2  force_law=Linear  k_contact=1e3  b_contact=100  pen_full_damp_F=1e-4  pen_exponent=1  custom_param_1=1  custom_param_2=1  friction_law=None  mu_kinetic=0.5  mu_static=0.7  v_thr=0.0001  vis_on=off  vis_opc_en=0  vis_len_plaBz=0.005  vis_clr=[0.9 0.2 0.2]  vis_opc=0.7
  Terminator{,1..6} (7 alike) : Terminator
  Transform Sensor : sm_lib/Frames and Transforms/Transform Sensor  MeasurementFrame=World  SenseAngle=off  SenseAxis=off  SenseAngle1=off  SenseAngle2=off  SenseAngle3=off  SenseQ=off  SenseR=off  SenseOmegaX=off  SenseOmegaY=off  SenseOmegaZ=off  SenseOmega1=off  SenseOmega2=off  SenseOmega3=off  SenseQDot=off  SenseRDot=off  SenseAlphaX=off  SenseAlphaY=off  SenseAlphaZ=off  SenseAlpha1=off  SenseAlpha2=off  SenseAlpha3=off  SenseQDDot=off  SenseRDDot=off  SenseX=on  SenseY=off  SenseZ=on  SenseRad=off  SenseAzim=off  SenseDist=off  SenseInc=off  SenseXDot=off  SenseYDot=off  SenseZDot=off  SenseRadDot=off  SenseAzimDot=off  SenseDistDot=off  SenseIncDot=off  SenseXDDot=off  SenseYDDot=off  SenseZDDot=off  SenseRadDDot=off  SenseAzimDDot=off  SenseDistDDot=off  SenseIncDDot=off
  XY Graph : simulink/Sinks/XY Graph  xmin=0  xmax=1.5  ymin=-1  ymax=1  st=-1
  L : PMIOPort  Side=Right
  Base : PMIOPort  Port=2  Side=Left
  Link_port : PMIOPort  Port=3  Side=Left
  Transform : PMIOPort  Port=4  Side=Left
  Ball_port : PMIOPort  Port=5  Side=Left
  wires:
  Sphere to Plane Force6/1 -> Terminator1/1
  Sphere to Plane Force3/1 -> Terminator5/1
  PS-Simulink Converter1/1 -> XY Graph/1
  Sphere to Plane Force2/1 -> Terminator4/1
  Sphere to Plane Force/1 -> Terminator6/1
  Sphere to Plane Force4/1 -> Terminator3/1
  Sphere to Plane Force5/1 -> Terminator/1
  PS-Simulink Converter2/1 -> XY Graph/2
  Sphere to Plane Force1/1 -> Terminator2/1
  connections:
  Sphere to Plane Force5/LConn1 -- Ball/RConn1 -- Ball_port/RConn1 -- Transform Sensor/RConn1 -- 6-DOF Joint/RConn1 -- Sphere to Plane Force6/LConn1 -- Sphere to Plane Force1/LConn1 -- Sphere to Plane Force2/LConn1 -- Sphere to Plane Force4/LConn1 -- Sphere to Plane Force3/LConn1
  Rigid Transform8/RConn1 -- Box_face1/RConn1 -- Rigid Transform11/LConn1 -- Rigid Transform9/LConn1 -- Rigid Transform12/LConn1 -- Rigid Transform15/LConn1
  Rigid Transform15/RConn1 -- Box_base/RConn1 -- Rigid Transform1/LConn1
  Sphere to Plane Force/LConn1 -- L/RConn1
  PS-Simulink Converter2/LConn1 -- Transform Sensor/RConn3
  Transform Sensor/LConn1 -- Transform/RConn1
  Sphere to Plane Force/RConn1 -- Box_base/LConn1
  Sphere to Plane Force1/RConn1 -- Box_face4/LConn1
  Rigid Transform8/LConn1 -- Link_port/RConn1
  Sphere to Plane Force3/RConn1 -- Box_face2/LConn1
  PS-Simulink Converter1/LConn1 -- Transform Sensor/RConn2
  Box_face3/RConn1 -- Rigid Transform9/RConn1
  Box_base/LConn2 -- Sphere to Plane Force6/RConn1
  Sphere to Plane Force4/RConn1 -- Box_face1/LConn1
  Sphere to Plane Force2/RConn1 -- Box_face3/LConn1
  Box_face4/RConn1 -- Rigid Transform12/RConn1
  Box_face2/RConn1 -- Rigid Transform11/RConn1
  6-DOF Joint/LConn1 -- Rigid Transform1/RConn1
  Sphere to Plane Force5/RConn1 -- Base/RConn1

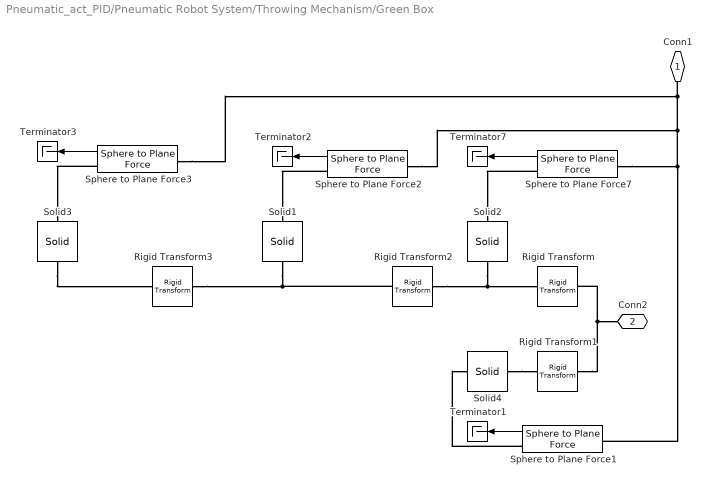
== system Pneumatic_act_PID/Pneumatic Robot System/Throwing Mechanism/Green Box ==
  Rigid Transform : sm_lib/Frames and Transforms/Rigid Transform  TranslationMethod=Cartesian  TranslationStandardOffset=0  TranslationLengthUnit=m  TranslationStandardAxis=+Z  TranslationCartesianOffset=[2.58 0 -0.15]  TranslationROffset=0  TranslationROffsetUnits=m  TranslationZOffset=0  TranslationZOffsetUnits=m  TranslationThetaOffset=0  TranslationThetaOffsetUnits=deg  RotationMethod=StandardAxis  RotationAngleUnits=deg  RotationStandardAxis=+Y  RotationAngle=90  RotationArbitraryAxis=[0 0 1]  FollAlignAxisA=+X  BaseAlignAxisA=+Y  FollAlignAxisB=+Y  BaseAlignAxisB=+Z  RotationSequenceAxes=FollowerAxes  RotationSequence=XYX  RotationSequenceAngles=[0 0 0]  RotationSequenceAnglesUnits=deg  RotationMatrix=[1 0 0; 0 1 0; 0 0 1]
  Rigid Transform1 : sm_lib/Frames and Transforms/Rigid Transform  TranslationMethod=Cartesian  TranslationStandardOffset=0  TranslationLengthUnit=m  TranslationStandardAxis=+Z  TranslationCartesianOffset=[2.28 0 -0.15]  TranslationROffset=0  TranslationROffsetUnits=m  TranslationZOffset=0  TranslationZOffsetUnits=m  TranslationThetaOffset=0  TranslationThetaOffsetUnits=deg  RotationMethod=StandardAxis  RotationAngleUnits=deg  RotationStandardAxis=+Y  RotationAngle=90  RotationArbitraryAxis=[0 0 1]  FollAlignAxisA=+X  BaseAlignAxisA=+Y  FollAlignAxisB=+Y  BaseAlignAxisB=+Z  RotationSequenceAxes=FollowerAxes  RotationSequence=XYX  RotationSequenceAngles=[0 0 0]  RotationSequenceAnglesUnits=deg  RotationMatrix=[1 0 0; 0 1 0; 0 0 1]
  Rigid Transform2 : sm_lib/Frames and Transforms/Rigid Transform  TranslationMethod=Cartesian  TranslationStandardOffset=0  TranslationLengthUnit=m  TranslationStandardAxis=+Z  TranslationCartesianOffset=[0 0.3/2 -0.3/2]  TranslationROffset=0  TranslationROffsetUnits=m  TranslationZOffset=0  TranslationZOffsetUnits=m  TranslationThetaOffset=0  TranslationThetaOffsetUnits=deg  RotationMethod=StandardAxis  RotationAngleUnits=deg  RotationStandardAxis=+X  RotationAngle=90  RotationArbitraryAxis=[0 0 1]  FollAlignAxisA=+X  BaseAlignAxisA=+Y  FollAlignAxisB=+Y  BaseAlignAxisB=+Z  RotationSequenceAxes=FollowerAxes  RotationSequence=XYX  RotationSequenceAngles=[0 0 0]  RotationSequenceAnglesUnits=deg  RotationMatrix=[1 0 0; 0 1 0; 0 0 1]
  Rigid Transform3 : sm_lib/Frames and Transforms/Rigid Transform  TranslationMethod=Cartesian  TranslationStandardOffset=0  TranslationLengthUnit=m  TranslationStandardAxis=+Z  TranslationCartesianOffset=[0 0 0.3]  TranslationROffset=0  TranslationROffsetUnits=m  TranslationZOffset=0  TranslationZOffsetUnits=m  TranslationThetaOffset=0  TranslationThetaOffsetUnits=deg  RotationMethod=None  RotationAngleUnits=deg  RotationStandardAxis=+X  RotationAngle=90  RotationArbitraryAxis=[0 0 1]  FollAlignAxisA=+X  BaseAlignAxisA=+Y  FollAlignAxisB=+Y  BaseAlignAxisB=+Z  RotationSequenceAxes=FollowerAxes  RotationSequence=XYX  RotationSequenceAngles=[0 0 0]  RotationSequenceAnglesUnits=deg  RotationMatrix=[1 0 0; 0 1 0; 0 0 1]
  Solid{1..4} (4 alike) : sm_lib/Body Elements/Solid  InertiaType=CalculateFromGeometry  Mass=1  MassUnits=kg  CenterOfMass=[0 0 0]  CenterOfMassUnits=m  MomentsOfInertia=[1 1 1]  MomentsOfInertiaUnits=kg*m^2  ProductsOfInertia=[0 0 0]  ProductsOfInertiaUnits=kg*m^2  BasedOnType=Density  Density=1000  DensityUnits=kg/m^3  DoExposeReferenceFrame=on  SerializedFrames=<Frames><Frame><Id>Frame1</Id><Value><Name>F1</Name><Origin><Source>ReferenceFrame</Source><FeatureName></FeatureName></Origin><PrimaryAxis><DefinedDirection>+Z</DefinedDirection><Source>ReferenceFrame</Source><SourceDirection>+Z</SourceDirection><FeatureName></FeatureName></PrimaryAxis><SecondaryAxis><DefinedDirection>+X</DefinedDirection><Source>ReferenceFrame</Source><SourceDirection>+X</SourceDirection><FeatureName></FeatureName></SecondaryAxis></Value></Frame></Frames>  GraphicType=FromGeometry  MarkerShape=Sphere  MarkerSize=10  GraphicVisPropType=SimpleVisualProperties  GraphicDiffuseColor=[0 0.8 0.4]  GraphicSpecularColor=[0.5 0.5 0.5 1.0]  GraphicAmbientColor=[0.15 0.15 0.15 1.0]  GraphicEmissiveColor=[0.0 0.0 0.0 1.0]  GraphicShininess=75  GraphicOpacity=0.3  GeometryShape=Brick  RectangleSize=[1 1]  RectangleSizeUnits=m  BrickDimensions=[box_yellow_length box_yellow_breadth box_yellow_height]  BrickDimensionUnits=m  CylinderRadius=1  CylinderRadiusUnits=m  CylinderLength=1  CylinderLengthUnits=m  SphereRadius=1  SphereRadiusUnits=m  EllipsoidRadii=[1 1 1]  EllipsoidRadiiUnits=m  ExtrusionCrossSection=[1 1; -1 1; -1 -1; 1 -1]  ExtrusionCrossSectionUnits=m  ExtrusionLength=1  ExtrusionLengthUnits=m  PolygonNumSides=3  PolygonOuterRadius=1  PolygonOuterRadiusUnits=m  ExtGeomFileType=STEP  ExtGeomFileUnits=m  RevolutionCrossSection=[1 1; 1 -1; 2 -1; 2 1]  RevolutionCrossSectionUnits=m  RevolutionExtent=Full  RevolutionAngle=180  RevolutionAngleUnits=deg
  Sphere to Plane Force{1..3,7} (4 alike) : Contact_Forces_Lib/3D/Sphere to Plane Force  sphere_rad=radius_ball  plane_lenx=box_yellow_length  plane_leny=box_yellow_breadth  plane_depth=box_yellow_height/2  force_law=Linear  k_contact=500  b_contact=100  pen_full_damp_F=1e-4  pen_exponent=1  custom_param_1=1  custom_param_2=1  friction_law=Stick-Slip Continuous  mu_kinetic=0.5  mu_static=0.7  v_thr=0.0001  vis_on=off  vis_opc_en=0  vis_len_plaBz=0.005  vis_clr=[0.9 0.2 0.2]  vis_opc=0.7
  Terminator{1..3,7} (4 alike) : Terminator
  Conn1 : PMIOPort  Side=Left
  Conn2 : PMIOPort  Port=2  Side=Right
  wires:
  Sphere to Plane Force3/1 -> Terminator3/1
  Sphere to Plane Force2/1 -> Terminator2/1
  Sphere to Plane Force1/1 -> Terminator1/1
  Sphere to Plane Force7/1 -> Terminator7/1
  connections:
  Sphere to Plane Force3/RConn1 -- Solid3/LConn1
  Sphere to Plane Force2/RConn1 -- Solid1/LConn1
  Sphere to Plane Force1/RConn1 -- Solid4/LConn1
  Solid4/RConn1 -- Rigid Transform1/RConn1
  Sphere to Plane Force7/RConn1 -- Solid2/LConn1
  Solid3/RConn1 -- Rigid Transform3/RConn1
  Rigid Transform/LConn1 -- Conn2/RConn1 -- Rigid Transform1/LConn1
  Solid1/RConn1 -- Rigid Transform3/LConn1 -- Rigid Transform2/RConn1
  Solid2/RConn1 -- Rigid Transform2/LConn1 -- Rigid Transform/RConn1
  Sphere to Plane Force1/LConn1 -- Sphere to Plane Force7/LConn1 -- Conn1/RConn1 -- Sphere to Plane Force3/LConn1 -- Sphere to Plane Force2/LConn1
